simulink model "OC_test"  (R2023b)
settings: Solver=VariableStepAuto  StartTime=0.0  StopTime=40  RelTol=1e-3
values from neighbouring files (symbols this model uses):
  Ra = 0.0096    [Start.m]    (also in Verification.m; cehck.m)
libraries: spsVoltageMeasurementLib x2, spsControlledVoltageSourceLib x1, spsDCMachineLib x1, spsGroundLib x1, sps_lib x1
settings Model: Creator=Hyeongmeen  LastModifiedBy=Hyeongmeen

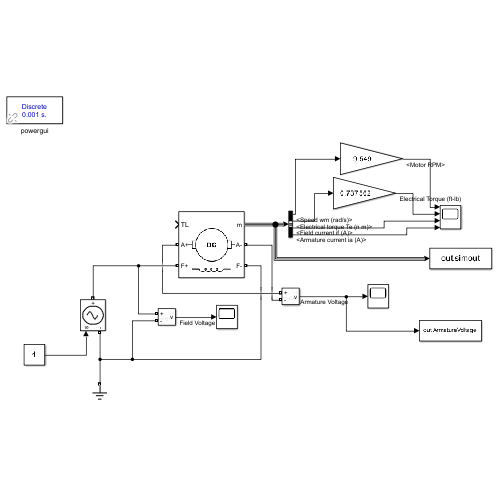
[thumbnail: Simulink's stored preview of the top-level diagram]
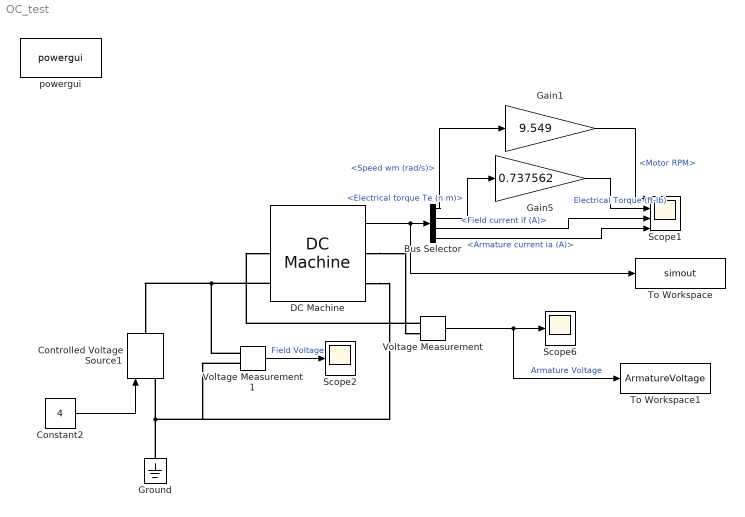
== system OC_test ==
  Bus Selector : BusSelector  OutputSignals=Speed wm (rad/s),Electrical torque Te (n m),Field current if (A),Armature current ia (A)
  Constant2 : Constant  Value=4
  Controlled Voltage Source1 : spsControlledVoltageSourceLib/Controlled Voltage Source  Initialize=on  Source_Type=DC  Amplitude=0  Phase=0  Frequency=0  Measurements=Voltage
  DC Machine : spsDCMachineLib/DC Machine  PresetModel=No  MechanicalLoad=Torque TL  FieldType=Wound  ShowDetailedParameters=on  MeasurementBus=off  RLa="[Ra  0.002]"  RLf=[0.0054 0.0125]  Laf=Laf  MachineConstant=Torque constant (N.m/A)  Ke=1.8  Kt=1.8  J=137  Bm=0  Tf=0  w0=w_initial  Ifinit=0  TsPowergui=0  TsBlock=-1
  Gain1 : Gain  Gain=9.549
  Gain5 : Gain  Gain=0.737562
  Ground : spsGroundLib/Ground  LConnTagsString=a
  Scope1 : Scope  NumInputPorts=4
  Scope2 : Scope
  Scope6 : Scope
  To Workspace : ToWorkspace  VariableName=simout  SaveFormat=Timeseries  SampleTime=-1
  To Workspace1 : ToWorkspace  VariableName=ArmatureVoltage  SaveFormat=Timeseries  SampleTime=-1
  Voltage Measurement : spsVoltageMeasurementLib/Voltage Measurement  PhasorSimulation=off  OutputType=Complex  PSBequivalent=0
  Voltage Measurement1 : spsVoltageMeasurementLib/Voltage Measurement  PhasorSimulation=off  OutputType=Complex  PSBequivalent=0
  powergui : sps_lib/powergui  Priority=1  SimulationMode=Discrete  SampleTime=1e-3  frequency=60  Iterations=50  frequencyindice=0  Pbase=100e6  ErrMax=1e-4  UnitsV=kV  UnitsW=MW  buscounter=0  FunctionMessages=off  echomessages=off  EnableUseOfTLC=off  CurrentSourceSwitches=off  DisableSnubberDevices=off  DisableRonSwitches=off  DisableVfSwitches=off  DisplayEquations=off  AutomaticDiscreteSolvers=off  SolverType=Tustin/Backward Euler (TBE)  Interpol=off  ExternalGateDelay=off  methode=off  Ts=100  x0status=blocks  SPID=on  SwTol=0  HookPort=off  NonlinearTolerance=1e-4  nMaxIteration=100  ContinueOnMaxIteration=off  RestoreLinks=warning  ResistiveCurrentMeasurement=off  Frange=[0:2:500]  Ylog=off  Xlog=on  ShowGrid=off  save=off  variable=ZData  structure=0  ZoomFFT=off  StartTime=0.0  cycles=1  DisplayStyle=1  fundamental=60  FreqAxis=off  MaxFrequency=1000  frequencyindicesteady=1  RmsSteady=1  display=off
  wires:
  Constant2/1 -> Controlled Voltage Source1/1
  Voltage Measurement/1 -> To Workspace1/1, Scope6/1  "Armature Voltage"
  DC Machine/1 -> To Workspace/1, Bus Selector/1
  Bus Selector/4 -> Scope1/4  "<Armature current ia (A)>"
  Gain5/1 -> Scope1/2  "Electrical Torque (ft-lb)"
  Bus Selector/2 -> Gain5/1  "<Electrical torque Te (n m)>"
  Gain1/1 -> Scope1/1  "<Motor RPM>"
  Bus Selector/1 -> Gain1/1  "<Speed wm (rad/s)>"
  Bus Selector/3 -> Scope1/3  "<Field current if (A)>"
  Voltage Measurement1/1 -> Scope2/1  "Field Voltage"
  connections:
  Ground/LConn1 -- Voltage Measurement1/LConn2 -- DC Machine/RConn2 -- Controlled Voltage Source1/LConn1
  DC Machine/LConn2 -- Voltage Measurement1/LConn1 -- Controlled Voltage Source1/RConn1
  Voltage Measurement/LConn1 -- DC Machine/LConn1
  DC Machine/RConn1 -- Voltage Measurement/LConn2
